simulink model "Quadcopter_nonlinear"  (R2020a)
settings: Solver=ode4  StartTime=0.0  StopTime=10  FixedStep=0.01  RelTol=1e-3
InitFcn:
  | close all
  | clc
  | Parameter_Modeling
  | ST=0.02;
  | angle_scale=.0109863;  % 1/91.0222
  | time_scale=.01;
  | QuadConstants
values from neighbouring files (symbols this model uses):
  AHRS = [45.076789856 45.076789856 45.076789856 45.076789856 45.076789856 45.076789856 45.076789856 45.076789856 45.076789856 45.076789856 45.076789856 45.076789856 ... (2002 elements, 1001x2)]    [Scenario_I.mat]    (also in Scenario_II.mat = [-33.5960998535 -33.5960998535 -33.5960998535 -33.5960998535)
undefined symbols (not defined in the file or in its folder): A1, A3, A5, AHRS_rate, magnitude
settings Model: Creator=Ali  LastModifiedBy=Ali
settings SolverCC: AlgebraicLoopSolver=LineSearch

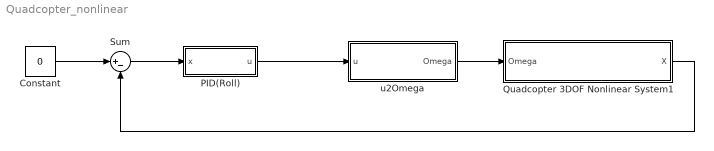
== system Quadcopter_nonlinear ==
  Constant : Constant  Value=0
  PID(Roll) : Subsystem
  Quadcopter 3DOF Nonlinear System1 : Subsystem  TreatAsAtomicUnit=on
  Sum : Sum  Inputs=|+-
  u2Omega : Subsystem
  wires:
  Quadcopter 3DOF Nonlinear System1/1(X) -> Sum/2
  u2Omega/1(Omega) -> Quadcopter 3DOF Nonlinear System1/1(Omega)
  Sum/1 -> PID(Roll)/1(x)
  PID(Roll)/1(u) -> u2Omega/1(u)
  Constant/1 -> Sum/1

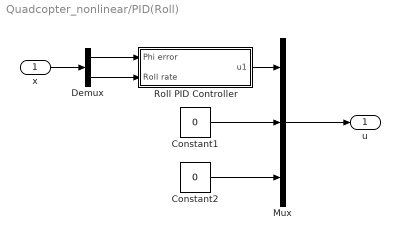
== system Quadcopter_nonlinear/PID(Roll) ==
  x : Inport
  Constant1 : Constant  Value=0
  Constant2 : Constant  Value=0
  Demux : Demux  Outputs=2
  Mux : Mux  Inputs=3
  Roll PID Controller : Subsystem  VariantControl=Choice
  u : Outport
  wires:
  Mux/1 -> u/1
  x/1 -> Demux/1
  Demux/2 -> Roll PID Controller/2(Roll rate)
  Constant2/1 -> Mux/3
  Demux/1 -> Roll PID Controller/1(Phi error)
  Roll PID Controller/1(u1) -> Mux/1
  Constant1/1 -> Mux/2

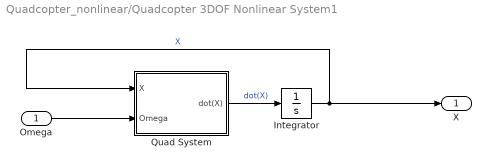
== system Quadcopter_nonlinear/Quadcopter 3DOF Nonlinear System1 ==
  Omega : Inport
  Integrator : Integrator  InitialCondition=[AHRS(1, 1)*pi/180 AHRS_rate(1, 1)*pi/180]
  Quad System : Subsystem
  X : Outport
  wires:
  Integrator/1 -> Quad System/1(X), X/1  "X"
  Quad System/1(dot(X)) -> Integrator/1  "dot(X)"
  Omega/1 -> Quad System/2(Omega)

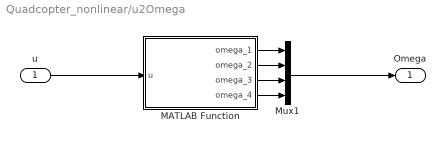
== system Quadcopter_nonlinear/u2Omega ==
  u : Inport
  MATLAB Function : MATLAB Function  TreatAsAtomicUnit=on
  Mux1 : Mux
  Omega : Outport
  wires:
  MATLAB Function/2(omega_2) -> Mux1/2
  u/1 -> MATLAB Function/1(u)
  MATLAB Function/3(omega_3) -> Mux1/3
  MATLAB Function/1(omega_1) -> Mux1/1
  MATLAB Function/4(omega_4) -> Mux1/4
  Mux1/1 -> Omega/1

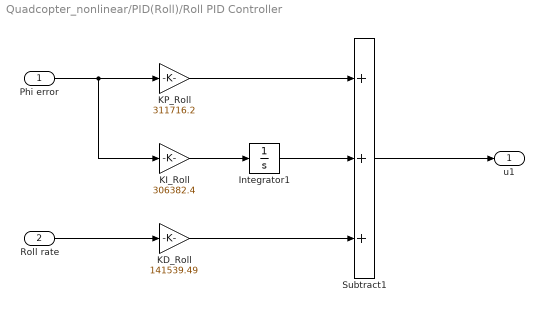
== system Quadcopter_nonlinear/PID(Roll)/Roll PID Controller ==
  Phi error : Inport
  Roll rate : Inport  Port=2
  Integrator1 : Integrator
  KD_Roll : Gain  Gain=141539.49
  KI_Roll : Gain  Gain=306382.4
  KP_Roll : Gain  Gain=311716.2
  Subtract1 : Sum  Inputs=+++
  u1 : Outport
  wires:
  Integrator1/1 -> Subtract1/2
  KI_Roll/1 -> Integrator1/1
  KD_Roll/1 -> Subtract1/3
  Subtract1/1 -> u1/1
  KP_Roll/1 -> Subtract1/1
  Roll rate/1 -> KD_Roll/1
  Phi error/1 -> KI_Roll/1, KP_Roll/1

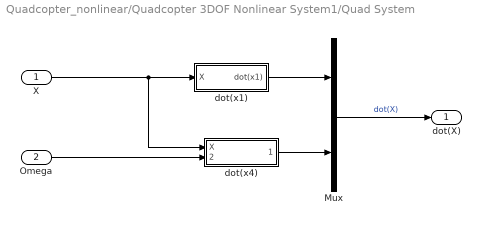
== system Quadcopter_nonlinear/Quadcopter 3DOF Nonlinear System1/Quad System ==
  X : Inport
  Omega : Inport  Port=2
  Mux : Mux  Inputs=2
  dot(x1) : Subsystem
  dot(x4) : Subsystem
  dot(X) : Outport
  wires:
  Mux/1 -> dot(X)/1  "dot(X)"
  X/1 -> dot(x4)/1(X), dot(x1)/1(X)
  Omega/1 -> dot(x4)/2(Omega)
  dot(x1)/1(dot(x1)) -> Mux/1
  dot(x4)/1(dot(x4)) -> Mux/2

== system Quadcopter_nonlinear/Quadcopter 3DOF Nonlinear System1/Quad System/dot(x1) ==
  X : Inport
  Subsystem1 : Subsystem
  dot(x1) : Outport
  wires:
  X/1 -> Subsystem1/1(X)  "X"
  Subsystem1/1(x4) -> dot(x1)/1

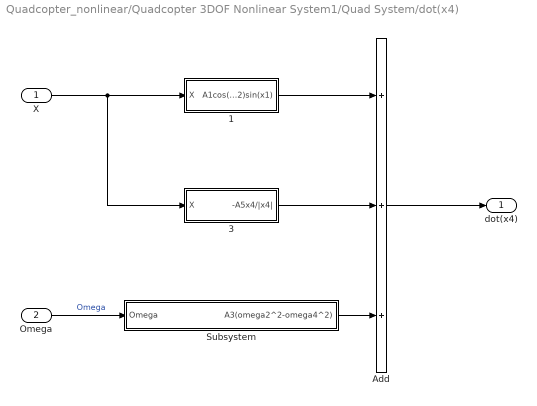
== system Quadcopter_nonlinear/Quadcopter 3DOF Nonlinear System1/Quad System/dot(x4) ==
  X : Inport
  Omega : Inport  Port=2
  1 : Subsystem
  3 : Subsystem
  Add : Sum  Inputs=+++
  Subsystem : Subsystem
  dot(x4) : Outport
  wires:
  Omega/1 -> Subsystem/1(Omega)  "Omega"
  Add/1 -> dot(x4)/1
  Subsystem/1(A3(omega2^2-omega4^2)) -> Add/3
  1/1(A1cos(x2)sin(x1)) -> Add/1
  3/1("-A5x4/|x4| ") -> Add/2
  X/1 -> 3/1(X), 1/1(X)

== system Quadcopter_nonlinear/Quadcopter 3DOF Nonlinear System1/Quad System/dot(x1)/Subsystem1 ==
  X : Inport
  Selector : Selector  InputPortWidth=2  IndexOptions=Index vector (dialog)  Indices=[2]  OutputSizes=1
  x4 : Outport
  wires:
  Selector/1 -> x4/1
  X/1 -> Selector/1

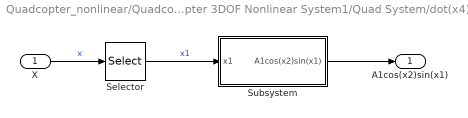
== system Quadcopter_nonlinear/Quadcopter 3DOF Nonlinear System1/Quad System/dot(x4)/1 ==
  X : Inport
  Selector : Selector  InputPortWidth=2  IndexOptions=Index vector (dialog)  Indices=[1]  OutputSizes=1
  Subsystem : Subsystem
  A1cos(x2)sin(x1) : Outport
  wires:
  Selector/1 -> Subsystem/1(x1)  "x1"
  Subsystem/1(A1cos(x2)sin(x1)) -> A1cos(x2)sin(x1)/1
  X/1 -> Selector/1  "x"

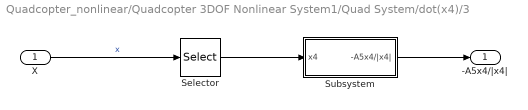
== system Quadcopter_nonlinear/Quadcopter 3DOF Nonlinear System1/Quad System/dot(x4)/3 ==
  X : Inport
  Selector : Selector  InputPortWidth=2  IndexOptions=Index vector (dialog)  Indices=[2]  OutputSizes=1
  Subsystem : Subsystem
  "-A5x4/|x4| " : Outport
  wires:
  Subsystem/1("-A5x4/|x4| ") -> "-A5x4/|x4| "/1
  X/1 -> Selector/1  "x"
  Selector/1 -> Subsystem/1(x4)

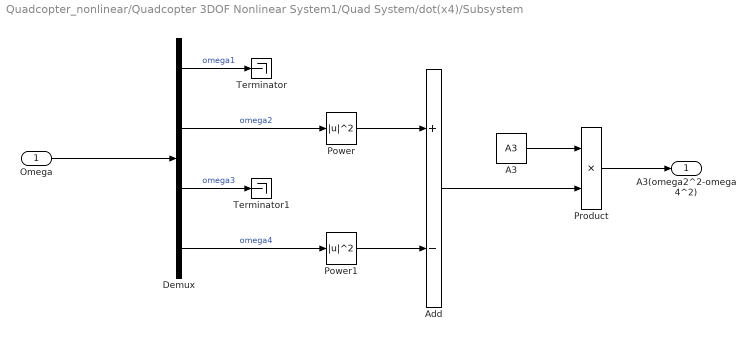
== system Quadcopter_nonlinear/Quadcopter 3DOF Nonlinear System1/Quad System/dot(x4)/Subsystem ==
  Omega : Inport
  A3 : Constant  Value=A3
  Add : Sum  Inputs=+-
  Demux : Demux
  Power : Math  Operator=magnitude^2  SaturateOnIntegerOverflow=on
  Power1 : Math  Operator=magnitude^2  SaturateOnIntegerOverflow=on
  Product : Product
  Terminator : Terminator
  Terminator1 : Terminator
  A3(omega2^2-omega4^2) : Outport
  wires:
  Product/1 -> A3(omega2^2-omega4^2)/1
  Power1/1 -> Add/2
  Demux/2 -> Power/1  "omega2"
  Demux/4 -> Power1/1  "omega4"
  Add/1 -> Product/2
  Power/1 -> Add/1
  A3/1 -> Product/1
  Omega/1 -> Demux/1
  Demux/3 -> Terminator1/1  "omega3"
  Demux/1 -> Terminator/1  "omega1"

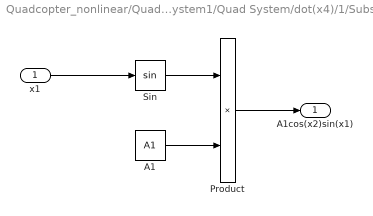
== system Quadcopter_nonlinear/Quadcopter 3DOF Nonlinear System1/Quad System/dot(x4)/1/Subsystem ==
  x1 : Inport
  A1 : Constant  Value=A1
  Product : Product
  Sin : Trigonometry
  A1cos(x2)sin(x1) : Outport
  wires:
  Sin/1 -> Product/1
  Product/1 -> A1cos(x2)sin(x1)/1
  x1/1 -> Sin/1
  A1/1 -> Product/2

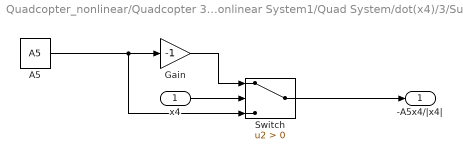
== system Quadcopter_nonlinear/Quadcopter 3DOF Nonlinear System1/Quad System/dot(x4)/3/Subsystem ==
  x4 : Inport
  A5 : Constant  Value=A5
  Gain : Gain  Gain=-1
  Switch : Switch  Criteria=u2 > Threshold
  "-A5x4/|x4| " : Outport
  wires:
  Switch/1 -> "-A5x4/|x4| "/1
  A5/1 -> Switch/3, Gain/1
  x4/1 -> Switch/2
  Gain/1 -> Switch/1

== matlab function Quadcopter_nonlinear/u2Omega/MATLAB Function ==
  data: u input size=3; omega_1 output size=1; omega_2 output size=1; omega_3 output size=1; omega_4 output size=1
function [omega_1, omega_2, omega_3, omega_4] = fcn(u)
u1 = u(1);
u2 = u(2);
u3 = u(3);
% control effort
u4 = ones(1, length(u1)) * 4 * rpm2rad_sec(2000)^2;
% calculate omega
if (u4 + u3 + 2 * u2) / 4 > 0
    omega_1 = sqrt((u4 + u3 + 2 * u2) / 4);
else
    omega_1 = 0;
end
if (u4 + u3 - 2 * u2) / 4 > 0
    omega_3 = sqrt((u4 + u3 - 2 * u2) / 4);
else
    omega_3 = 0;
end
if (u4 - u3 + 2 * u1) / 4 > 0
    omega_2 = sqrt((u4 - u3 + 2 * u1) / 4);
else
    omega_2 = 0;
end
if (u4 - u3 - 2 * u1) / 4 > 0
    omega_4 = sqrt((u4 - u3 - 2 * u1) / 4);
else
    omega_4 = 0;
end
end
%% functions
% rpm to rad/sec
function rad = rpm2rad_sec(rpm)
rad = rpm / 60 * 2 * pi;
end
